simulink model "dsm_l2_sim_deci_cic_HDLgeneration"  (R2025b)
settings: Solver=FixedStepDiscrete  StartTime=0.0  StopTime=1024  RelTol=1e-3  AbsTol=1e-6
values from neighbouring files (symbols this model uses):
  a1 = a(1)    [dsm_l1.m]    (also in dsm_o2_Simulink_HDLgeneration.m; dsm_o2_Simulink_compare.m; dsm_o2_Simulink_decimation.m; hodiewindow.m = 0.985371192726)
  a2 = a(2)    [dsm_l1.m]    (also in dsm_o2_Simulink_HDLgeneration.m; dsm_o2_Simulink_compare.m; dsm_o2_Simulink_decimation.m; hodiewindow.m = 0.49603771622)
  b1 = b(1)    [dsm_l1.m]    (also in dsm_o2_Simulink_HDLgeneration.m; dsm_o2_Simulink_compare.m; dsm_o2_Simulink_decimation.m; my_dsm_v1.m)
  c1 = c(1)    [dsm_l1.m]    (also in dsm_o2_Simulink_HDLgeneration.m; dsm_o2_Simulink_compare.m; dsm_o2_Simulink_decimation.m; my_dsm_v1.m)
  c2 = c(2)    [dsm_l1.m]    (also in dsm_o2_Simulink_HDLgeneration.m; dsm_o2_Simulink_compare.m; dsm_o2_Simulink_decimation.m; my_dsm_v1.m)
  DCFnum = Hdcf.Numerator    [decimation_filters.m]    (also in dsm_decimator_sim.m; dsm_l2_delsig_scmod2.m; dsm_o2_Simulink_HDLgeneration.m; dsm_o2_Simulink_decimation.m)
  fs = 1e6    (= 1000000)    [decimation_filters.m]    (also in dsm_decimator_sim.m; dsm_l1.m = 1; dsm_l1_dither.m = 1; dsm_l1_ntf.m = 1)
  HBF1num = firhalfband(HBF1taps, 0.25)    [decimation_filters.m]    (also in dsm_decimator_sim.m; dsm_l2_delsig_scmod2.m; dsm_o2_Simulink_HDLgeneration.m; dsm_o2_Simulink_decimation.m)
  HBF2num = firhalfband(HBF2taps, 0.25)    [decimation_filters.m]    (also in dsm_decimator_sim.m; dsm_l2_delsig_scmod2.m; dsm_o2_Simulink_HDLgeneration.m; dsm_o2_Simulink_decimation.m)
  Ts = 1/fs    (= 1e-06)    [dsm_decimator_sim.m]    (also in dsm_l1.m = 1; dsm_l1_dither.m = 1; dsm_l1_ntf.m = 1; dsm_l1_sin.m = 1)
undefined symbols (not defined in the file or in its folder): dspblkCoreblockFVToolHelper, gcbh
libraries: dsphdlfiltering2 x4, dspsrcs4 x1
settings Model: DataTypeOverride=Off  Creator=mimeiners  LastModifiedBy=korvo
settings SolverCC: AutoScaleAbsTol=off  AlgebraicLoopSolver=TrustRegion
settings DataIOCC: ExternalInput=[]  SaveFormat=Array  ReturnWorkspaceOutputs=off  SignalLoggingName=sigsOut
settings OptimizationCC: BlockReduction=off  BooleanDataType=off  ConditionallyExecuteInputs=off  DefaultParameterBehavior=Inlined  InheritOutputTypeSmallerThanSingle=on  ReuseModelBlockBuffer=off
settings DebuggingCC: AlgebraicLoopMsg=error  SaveWithParameterizedLinksMsg=none  UnderspecifiedInitializationDetection=Classic  MergeDetectMultiDrivingBlocksExec=none  SignalResolutionControl=TryResolveAllWithWarning  MultiTaskDSMMsg=warning  MultiTaskCondExecSysMsg=none  SingleTaskRateTransMsg=error  UnconnectedInputMsg=warning  UnconnectedOutputMsg=warning  UnconnectedLineMsg=warning  ArithmeticOperatorsInVariantConditions=warning
settings HardwareCC: ProdBitPerPointer=32.0  ProdBitPerSizeT=32.0  ProdBitPerPtrDiffT=32.0  ProdLargestAtomicFloat=None  ProdIntDivRoundTo=Undefined  ProdEndianess=Unspecified  ProdWordSize=32.0  ProdHWDeviceType=ASIC/FPGA->ASIC/FPGA  TargetBitPerPointer=64.0  TargetBitPerSizeT=64.0  TargetBitPerPtrDiffT=64.0  TargetLongLongMode=on  TargetIntDivRoundTo=Zero  TargetEndianess=LittleEndian  TargetWordSize=64.0  TargetHWDeviceType=Custom Processor->MATLAB Host Computer  TargetUnknown=on  ProdEqTarget=off
settings ModelReferenceCC: EnableRefExpFcnMdlSchedulingChecks=on  PropagateSignalLabelsOutOfModel=off
settings SFSimCC: SimUseLocalCustomCode=off  CustomCodeUndefinedFunction=UseInterfaceOnly
settings RTWCC: TemplateMakefile=grt_vc.tmf  RTWUseLocalCustomCode=off  GPUComputeCapability=3.5  DLArmComputeVersion=19.05
settings GRTTargetCC: TargetLangStandard=C89/C90 (ANSI)  CombineOutputUpdateFcns=off  GRTInterface=on
settings ConfigComp: CovMetricSettings=dw  CovSaveCumulativeToWorkspaceVar=on  CovSaveSingleToWorkspaceVar=on  CovExternalEMLEnable=off

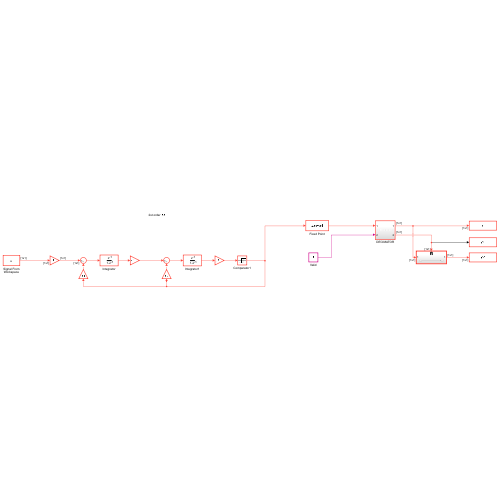
[thumbnail: Simulink's stored preview of the top-level diagram]
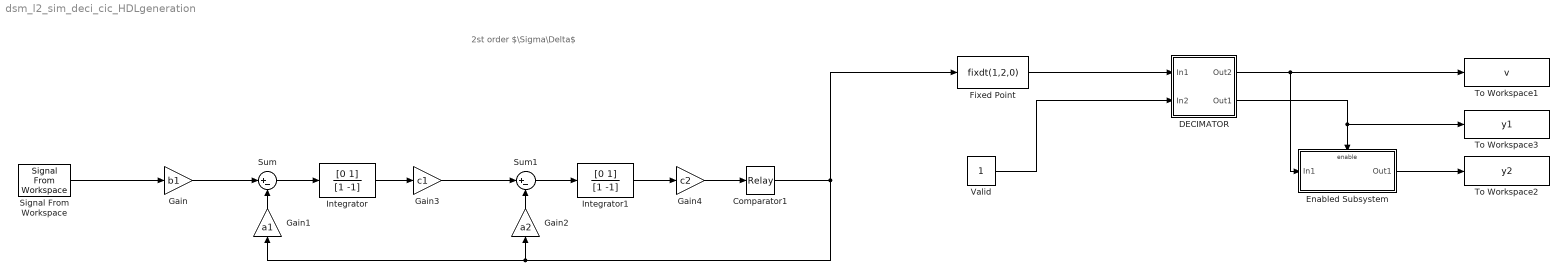
== system dsm_l2_sim_deci_cic_HDLgeneration ==
  note: 2st order $\Sigma\Delta$
  Comparator1 : Relay  OffOutputValue=-1
  DECIMATOR : Subsystem
  Enabled Subsystem : Subsystem  TreatAsAtomicUnit=on
  Fixed Point : DataTypeConversion  OutDataTypeStr=fixdt(1,2,0)  RndMeth=Nearest  SaturateOnIntegerOverflow=off
  Gain : Gain  Gain=b1
  Gain1 : Gain  Gain=a1
  Gain2 : Gain  Gain=a2
  Gain3 : Gain  Gain=c1
  Gain4 : Gain  Gain=c2
  Integrator : DiscreteFilter  LoadFcn=dspblkCoreblockFVToolHelper(gcbh,'load');  Numerator=[0 1]  Denominator=[1 -1]  SampleTime=Ts
      settings: CopyFcn=dspblkCoreblockFVToolHelper(gcbh,'copy');  DeleteFcn=dspblkCoreblockFVToolHelper(gcbh,'close');  ModelCloseFcn=dspblkCoreblockFVToolHelper(gcbh,'close');  PreSaveFcn=dspblkCoreblockFVToolHelper(gcbh,'presave');  PostSaveFcn=dspblkCoreblockFVToolHelper(gcbh,'postsave');  CloseFcn=dspblkCoreblockFVToolHelper(gcbh,'close');
  Integrator1 : DiscreteFilter  LoadFcn=dspblkCoreblockFVToolHelper(gcbh,'load');  Numerator=[0 1]  Denominator=[1 -1]  SampleTime=Ts
      settings: CopyFcn=dspblkCoreblockFVToolHelper(gcbh,'copy');  DeleteFcn=dspblkCoreblockFVToolHelper(gcbh,'close');  ModelCloseFcn=dspblkCoreblockFVToolHelper(gcbh,'close');  PreSaveFcn=dspblkCoreblockFVToolHelper(gcbh,'presave');  PostSaveFcn=dspblkCoreblockFVToolHelper(gcbh,'postsave');  CloseFcn=dspblkCoreblockFVToolHelper(gcbh,'close');
  Signal From Workspace : dspsrcs4/Signal From Workspace  X=u  Ts=1/fs  nsamps=1  OutputAfterFinalValue=Setting to zero  ignoreOrWarnInputAndFrameLengths=off  OutputFrames=off
  Sum : Sum  Inputs=|+-  InputSameDT=on  SaturateOnIntegerOverflow=on  OutDataTypeStr=Inherit: Same as first input
  Sum1 : Sum  Inputs=|+-  InputSameDT=on  SaturateOnIntegerOverflow=on  OutDataTypeStr=Inherit: Same as first input
  To Workspace1 : ToWorkspace  VariableName=v  SampleTime=-1
      settings: Save2DSignal=2-D array (concatenate along first dimension)
  To Workspace2 : ToWorkspace  VariableName=y2  SampleTime=-1
      settings: Save2DSignal=2-D array (concatenate along first dimension)
  To Workspace3 : ToWorkspace  VariableName=y1  SampleTime=-1
      settings: Save2DSignal=2-D array (concatenate along first dimension)
  Valid : Constant  OutDataTypeStr=boolean
  wires:
  Sum/1 -> Integrator/1
  Integrator/1 -> Gain3/1
  Signal From Workspace/1 -> Gain/1
  Gain3/1 -> Sum1/1
  Sum1/1 -> Integrator1/1
  Integrator1/1 -> Gain4/1
  Gain/1 -> Sum/1
  Gain1/1 -> Sum/2
  Gain2/1 -> Sum1/2
  Gain4/1 -> Comparator1/1
  Comparator1/1 -> Fixed Point/1, Gain1/1, Gain2/1
  Fixed Point/1 -> DECIMATOR/1(In1)
  DECIMATOR/1(Out2) -> Enabled Subsystem/1(In1), To Workspace1/1
  Valid/1 -> DECIMATOR/2(In2)
  DECIMATOR/2(Out1) -> To Workspace3/1, Enabled Subsystem/Enable
  Enabled Subsystem/1(Out1) -> To Workspace2/1

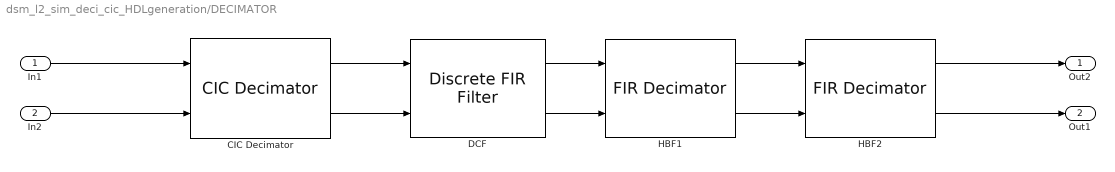
== system dsm_l2_sim_deci_cic_HDLgeneration/DECIMATOR ==
  In1 : Inport
  In2 : Inport  Port=2
  CIC Decimator : dsphdlfiltering2/CIC Decimator  DecimationSource=Property  DecimationFactor=Nsinc  MaxDecimationFactor=2  DifferentialDelay=1  NumSections=3  GainCorrection=on  SimulateUsing=Code generation  OutputDataType=Minimum section word lengths  OutputWordLength=16  ResetInputPort=off  HDLGlobalReset=on
  DCF : dsphdlfiltering2/Discrete FIR Filter  NumeratorSource=Property  Numerator=DCFnum  NumeratorPrototype=[]  FilterStructure=Direct form systolic  SerializationOption=Minimum number of cycles between valid input samples  NumCycles=2  NumberOfMultipliers=2  SimulateUsing=Code generation  roundingMode=Floor  overflowMode=off  CoefficientsDataTypeStr=Inherit: Same word length as input  ResetInputPort=off  HDLGlobalReset=on  CoeffMultiplier=Multiplier  UseMultForPow2Coeff=on  FrameInputSymmOptim=on
  HBF1 : dsphdlfiltering2/FIR Decimator  NumeratorSource=Property  Numerator=HBF1num  NumeratorPrototype=[]  FilterStructure=Direct form systolic  DecimationFactor=2  NumCycles=1  OptimizeSymmCoeff=on  SimulateUsing=Code generation  roundingMode=Floor  overflowMode=off  CoefficientsDataTypeStr=Inherit: Same word length as input  ResetInputPort=off  HDLGlobalReset=on
  HBF2 : dsphdlfiltering2/FIR Decimator  NumeratorSource=Property  Numerator=HBF2num  NumeratorPrototype=[]  FilterStructure=Direct form systolic  DecimationFactor=2  NumCycles=1  OptimizeSymmCoeff=on  SimulateUsing=Code generation  roundingMode=Floor  overflowMode=off  CoefficientsDataTypeStr=Inherit: Same word length as input  ResetInputPort=off  HDLGlobalReset=on
  Out2 : Outport
  Out1 : Outport  Port=2
  wires:
  CIC Decimator/1 -> DCF/1
  HBF1/2 -> HBF2/2
  CIC Decimator/2 -> DCF/2
  In1/1 -> CIC Decimator/1
  In2/1 -> CIC Decimator/2
  DCF/1 -> HBF1/1
  DCF/2 -> HBF1/2
  HBF1/1 -> HBF2/1
  HBF2/1 -> Out2/1
  HBF2/2 -> Out1/1

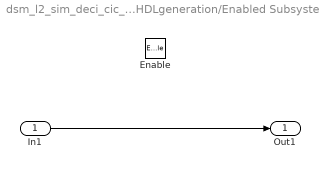
== system dsm_l2_sim_deci_cic_HDLgeneration/Enabled Subsystem ==
  In1 : Inport
  Enable : EnablePort
  Out1 : Outport
  wires:
  In1/1 -> Out1/1
